simulink model "X31dynamics_03_controller_NDI_MG"  (R2014b)
settings: Solver=ode45  StartTime=0.0  StopTime=30  FixedStep=0.01  RelTol=1e-3
InitFcn:
  | X31dynamics_03_controller_NDI_init
values from neighbouring files (symbols this model uses):
  X31_controller = evalin('base','X31_controller')    [X31dynamics_03_controller_MG_iter_3_2_9_10.m]
undefined symbols (not defined in the file or in its folder): sigbuilder_block, X31_initC, X31_MnvrGen
libraries: simulink x17, QuaternionLib x3
(part 1 of 2)
settings Model: Creator=Ewing  LastModifiedBy=5909
settings SolverCC: AlgebraicLoopSolver=LineSearch
settings DataIOCC: SaveOutput=off  SaveTime=off
settings OptimizationCC: InlineParams=on  InlineInvariantSignals=on  EfficientFloat2IntCast=on
settings DebuggingCC: UnderspecifiedInitializationDetection=Classic  MergeDetectMultiDrivingBlocksExec=none  UniqueDataStoreMsg=error  StateNameClashWarn=warning
settings ModelReferenceCC: ModelReferencePassRootInputsByReference=off

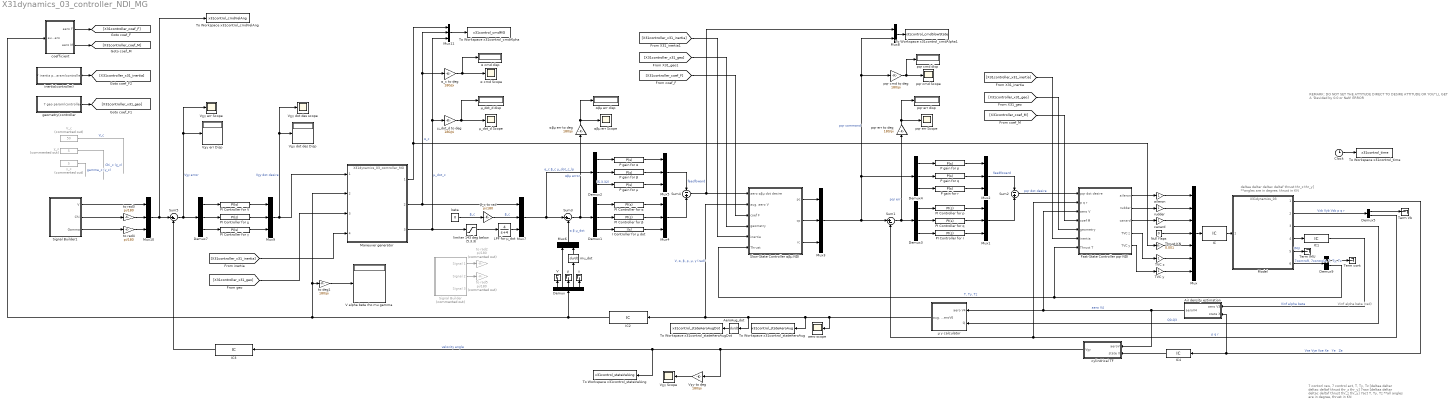
== system X31dynamics_03_controller_NDI_MG ==
  note: REMARK: DO NOT SET THE ATTITUDE DIRECT TO DESIRE ATTITUDE
      | OR YOU"LL GET A 'Devided by 0.0 or NaN' ERROR
  note: deltaa deltar deltac deltaf thrust thr_z thr_y]
      | **angles are in degree, thrust in KN
  note: Vinf alpha beta (rad)
  note: 7 contorl raw, 7 control act, T, Ty, Tz
      | [deltaa deltar deltac deltaf thrust thr_z thr_y] 7raw
      | [deltaa deltar deltac deltaf thrust thr_z thr_y] 7act
      | T, Ty, Tz
      | **all angles are in degree, thrust in KN
  AeroAug_dot : Derivative
  Air density estimation : Subsystem
  Clock : Clock
  Demux : Demux  Outputs=[1 2 1 1 1]
  Demux{1..4,7} (5 alike) : Demux  Outputs=3
  Demux5 : Demux  Outputs=[3 3]
  Demux9 : Demux  Outputs=[14 3]
  Fast-State Controller pqr NDI : Subsystem
  I Controller for μ dot : simulink/Continuous/PID Controller  Controller=I  TimeDomain=Continuous-time  SampleTime=-1  IntegratorMethod=Forward Euler  FilterMethod=Forward Euler  Form=Parallel  P=1  I=X31_controller.gains.slow_st.mu_dot.I_gain  D=0  N=100  InitialConditionSource=internal  InitialConditionForIntegrator=0  InitialConditionForFilter=0  ExternalReset=none  LimitOutput=off  UpperSaturationLimit=inf  LowerSaturationLimit=-inf  LinearizeAsGain=on  AntiWindupMode=none  Kb=1  TrackingMode=off  Kt=1  PParamMin=[]  PParamMax=[]  IParamMin=[]  IParamMax=[]  DParamMin=[]  DParamMax=[]  NParamMin=[]  NParamMax=[]  KbParamMin=[]  KbParamMax=[]  KtParamMin=[]  KtParamMax=[]  POutMin=[]  POutMax=[]  IOutMin=[]  IOutMax=[]  DOutMin=[]  DOutMax=[]  NOutMin=[]  NOutMax=[]  KbOutMin=[]  KbOutMax=[]  KtOutMin=[]  KtOutMax=[]  IntegratorOutMin=[]  IntegratorOutMax=[]  FilterOutMin=[]  FilterOutMax=[]  SumOutMin=[]  SumOutMax=[]  SumI1OutMin=[]  SumI1OutMax=[]  SumI2OutMin=[]  SumI2OutMax=[]  SumI3OutMin=[]  SumI3OutMax=[]  SumDOutMin=[]  SumDOutMax=[]  SaturationOutMin=[]  SaturationOutMax=[]  IntegratorContinuousStateAttributes=''  IntegratorStateMustResolveToSignalObject=off  IntegratorRTWStateStorageClass=Auto  FilterContinuousStateAttributes=''  FilterStateMustResolveToSignalObject=off  FilterRTWStateStorageClass=Auto  DifferentiatorICPrevScaledInput=0  DifferentiatorOutMin=[]  DifferentiatorOutMax=[]  UseFilter=on
  IC : InitialCondition  Value=[ 0.0001 0.0001 0.0001 0.0001 X31_initC.thrust 0.0001 0.0001]
  IC1 : InitialCondition  Value=[50 0.01 0.01]
  IC2 : InitialCondition  Value=[50 5 0 1.23 0 0]
  IC3 : InitialCondition  Value=[50 0 0]
  IC4 : InitialCondition  Value=[50 0 0 0.1 0.1 -0.1]
  LPF for μ_dot : TransferFcn  Numerator=[4]  Denominator=[1 4]
  Maneuver generator : ModelReference  ModelNameDialog=X31dynamics_03_controller_MG.slx  SimulationMode=Normal  ModelReferenceVersion=1.4  CopyOfModelName=X31dynamics_03_controller_MG.slx  DefaultDataLogging=on
  Model : ModelReference  ModelNameDialog=X31dynamics_03.slx  SimulationMode=Normal  ModelReferenceVersion=1.305  CopyOfModelName=X31dynamics_03.slx  DefaultDataLogging=on
  Mux : Mux  Inputs=7
  Mux{1..5,7,9..11} (9 alike) : Mux  Inputs=3
  Mux6 : Mux  Inputs=2
  Mux8 : Mux  Inputs=2
  Null flaps : Constant  Value=0
  P gain for p : simulink/Continuous/PID Controller  Controller=P  TimeDomain=Continuous-time  SampleTime=-1  IntegratorMethod=Forward Euler  FilterMethod=Forward Euler  Form=Parallel  P=X31_controller.gains.fast_st.p.ff_gain  I=1  D=0  N=100  InitialConditionSource=internal  InitialConditionForIntegrator=0  InitialConditionForFilter=0  ExternalReset=none  LimitOutput=off  UpperSaturationLimit=inf  LowerSaturationLimit=-inf  LinearizeAsGain=on  AntiWindupMode=none  Kb=1  TrackingMode=off  Kt=1  PParamMin=[]  PParamMax=[]  IParamMin=[]  IParamMax=[]  DParamMin=[]  DParamMax=[]  NParamMin=[]  NParamMax=[]  KbParamMin=[]  KbParamMax=[]  KtParamMin=[]  KtParamMax=[]  POutMin=[]  POutMax=[]  IOutMin=[]  IOutMax=[]  DOutMin=[]  DOutMax=[]  NOutMin=[]  NOutMax=[]  KbOutMin=[]  KbOutMax=[]  KtOutMin=[]  KtOutMax=[]  IntegratorOutMin=[]  IntegratorOutMax=[]  FilterOutMin=[]  FilterOutMax=[]  SumOutMin=[]  SumOutMax=[]  SumI1OutMin=[]  SumI1OutMax=[]  SumI2OutMin=[]  SumI2OutMax=[]  SumI3OutMin=[]  SumI3OutMax=[]  SumDOutMin=[]  SumDOutMax=[]  SaturationOutMin=[]  SaturationOutMax=[]  IntegratorContinuousStateAttributes=''  IntegratorStateMustResolveToSignalObject=off  IntegratorRTWStateStorageClass=Auto  FilterContinuousStateAttributes=''  FilterStateMustResolveToSignalObject=off  FilterRTWStateStorageClass=Auto  DifferentiatorICPrevScaledInput=0  DifferentiatorOutMin=[]  DifferentiatorOutMax=[]  UseFilter=on
  P gain for q : simulink/Continuous/PID Controller  Controller=P  TimeDomain=Continuous-time  SampleTime=-1  IntegratorMethod=Forward Euler  FilterMethod=Forward Euler  Form=Parallel  P=X31_controller.gains.fast_st.q.ff_gain  I=1  D=0  N=100  InitialConditionSource=internal  InitialConditionForIntegrator=0  InitialConditionForFilter=0  ExternalReset=none  LimitOutput=off  UpperSaturationLimit=inf  LowerSaturationLimit=-inf  LinearizeAsGain=on  AntiWindupMode=none  Kb=1  TrackingMode=off  Kt=1  PParamMin=[]  PParamMax=[]  IParamMin=[]  IParamMax=[]  DParamMin=[]  DParamMax=[]  NParamMin=[]  NParamMax=[]  KbParamMin=[]  KbParamMax=[]  KtParamMin=[]  KtParamMax=[]  POutMin=[]  POutMax=[]  IOutMin=[]  IOutMax=[]  DOutMin=[]  DOutMax=[]  NOutMin=[]  NOutMax=[]  KbOutMin=[]  KbOutMax=[]  KtOutMin=[]  KtOutMax=[]  IntegratorOutMin=[]  IntegratorOutMax=[]  FilterOutMin=[]  FilterOutMax=[]  SumOutMin=[]  SumOutMax=[]  SumI1OutMin=[]  SumI1OutMax=[]  SumI2OutMin=[]  SumI2OutMax=[]  SumI3OutMin=[]  SumI3OutMax=[]  SumDOutMin=[]  SumDOutMax=[]  SaturationOutMin=[]  SaturationOutMax=[]  IntegratorContinuousStateAttributes=''  IntegratorStateMustResolveToSignalObject=off  IntegratorRTWStateStorageClass=Auto  FilterContinuousStateAttributes=''  FilterStateMustResolveToSignalObject=off  FilterRTWStateStorageClass=Auto  DifferentiatorICPrevScaledInput=0  DifferentiatorOutMin=[]  DifferentiatorOutMax=[]  UseFilter=on
  P gain for r : simulink/Continuous/PID Controller  Controller=P  TimeDomain=Continuous-time  SampleTime=-1  IntegratorMethod=Forward Euler  FilterMethod=Forward Euler  Form=Parallel  P=X31_controller.gains.fast_st.r.ff_gain  I=1  D=0  N=100  InitialConditionSource=internal  InitialConditionForIntegrator=0  InitialConditionForFilter=0  ExternalReset=none  LimitOutput=off  UpperSaturationLimit=inf  LowerSaturationLimit=-inf  LinearizeAsGain=on  AntiWindupMode=none  Kb=1  TrackingMode=off  Kt=1  PParamMin=[]  PParamMax=[]  IParamMin=[]  IParamMax=[]  DParamMin=[]  DParamMax=[]  NParamMin=[]  NParamMax=[]  KbParamMin=[]  KbParamMax=[]  KtParamMin=[]  KtParamMax=[]  POutMin=[]  POutMax=[]  IOutMin=[]  IOutMax=[]  DOutMin=[]  DOutMax=[]  NOutMin=[]  NOutMax=[]  KbOutMin=[]  KbOutMax=[]  KtOutMin=[]  KtOutMax=[]  IntegratorOutMin=[]  IntegratorOutMax=[]  FilterOutMin=[]  FilterOutMax=[]  SumOutMin=[]  SumOutMax=[]  SumI1OutMin=[]  SumI1OutMax=[]  SumI2OutMin=[]  SumI2OutMax=[]  SumI3OutMin=[]  SumI3OutMax=[]  SumDOutMin=[]  SumDOutMax=[]  SaturationOutMin=[]  SaturationOutMax=[]  IntegratorContinuousStateAttributes=''  IntegratorStateMustResolveToSignalObject=off  IntegratorRTWStateStorageClass=Auto  FilterContinuousStateAttributes=''  FilterStateMustResolveToSignalObject=off  FilterRTWStateStorageClass=Auto  DifferentiatorICPrevScaledInput=0  DifferentiatorOutMin=[]  DifferentiatorOutMax=[]  UseFilter=on
  P gain for α : simulink/Continuous/PID Controller  Controller=P  TimeDomain=Continuous-time  SampleTime=-1  IntegratorMethod=Forward Euler  FilterMethod=Forward Euler  Form=Parallel  P=X31_controller.gains.slow_st.alpha.ff_gain  I=1  D=0  N=100  InitialConditionSource=internal  InitialConditionForIntegrator=0  InitialConditionForFilter=0  ExternalReset=none  LimitOutput=off  UpperSaturationLimit=inf  LowerSaturationLimit=-inf  LinearizeAsGain=on  AntiWindupMode=none  Kb=1  TrackingMode=off  Kt=1  PParamMin=[]  PParamMax=[]  IParamMin=[]  IParamMax=[]  DParamMin=[]  DParamMax=[]  NParamMin=[]  NParamMax=[]  KbParamMin=[]  KbParamMax=[]  KtParamMin=[]  KtParamMax=[]  POutMin=[]  POutMax=[]  IOutMin=[]  IOutMax=[]  DOutMin=[]  DOutMax=[]  NOutMin=[]  NOutMax=[]  KbOutMin=[]  KbOutMax=[]  KtOutMin=[]  KtOutMax=[]  IntegratorOutMin=[]  IntegratorOutMax=[]  FilterOutMin=[]  FilterOutMax=[]  SumOutMin=[]  SumOutMax=[]  SumI1OutMin=[]  SumI1OutMax=[]  SumI2OutMin=[]  SumI2OutMax=[]  SumI3OutMin=[]  SumI3OutMax=[]  SumDOutMin=[]  SumDOutMax=[]  SaturationOutMin=[]  SaturationOutMax=[]  IntegratorContinuousStateAttributes=''  IntegratorStateMustResolveToSignalObject=off  IntegratorRTWStateStorageClass=Auto  FilterContinuousStateAttributes=''  FilterStateMustResolveToSignalObject=off  FilterRTWStateStorageClass=Auto  DifferentiatorICPrevScaledInput=0  DifferentiatorOutMin=[]  DifferentiatorOutMax=[]  UseFilter=on
  P gain for β : simulink/Continuous/PID Controller  Controller=P  TimeDomain=Continuous-time  SampleTime=-1  IntegratorMethod=Forward Euler  FilterMethod=Forward Euler  Form=Parallel  P=X31_controller.gains.slow_st.beta.ff_gain  I=1  D=0  N=100  InitialConditionSource=internal  InitialConditionForIntegrator=0  InitialConditionForFilter=0  ExternalReset=none  LimitOutput=off  UpperSaturationLimit=inf  LowerSaturationLimit=-inf  LinearizeAsGain=on  AntiWindupMode=none  Kb=1  TrackingMode=off  Kt=1  PParamMin=[]  PParamMax=[]  IParamMin=[]  IParamMax=[]  DParamMin=[]  DParamMax=[]  NParamMin=[]  NParamMax=[]  KbParamMin=[]  KbParamMax=[]  KtParamMin=[]  KtParamMax=[]  POutMin=[]  POutMax=[]  IOutMin=[]  IOutMax=[]  DOutMin=[]  DOutMax=[]  NOutMin=[]  NOutMax=[]  KbOutMin=[]  KbOutMax=[]  KtOutMin=[]  KtOutMax=[]  IntegratorOutMin=[]  IntegratorOutMax=[]  FilterOutMin=[]  FilterOutMax=[]  SumOutMin=[]  SumOutMax=[]  SumI1OutMin=[]  SumI1OutMax=[]  SumI2OutMin=[]  SumI2OutMax=[]  SumI3OutMin=[]  SumI3OutMax=[]  SumDOutMin=[]  SumDOutMax=[]  SaturationOutMin=[]  SaturationOutMax=[]  IntegratorContinuousStateAttributes=''  IntegratorStateMustResolveToSignalObject=off  IntegratorRTWStateStorageClass=Auto  FilterContinuousStateAttributes=''  FilterStateMustResolveToSignalObject=off  FilterRTWStateStorageClass=Auto  DifferentiatorICPrevScaledInput=0  DifferentiatorOutMin=[]  DifferentiatorOutMax=[]  UseFilter=on
  P gain for μ : simulink/Continuous/PID Controller  Controller=P  TimeDomain=Continuous-time  SampleTime=-1  IntegratorMethod=Forward Euler  FilterMethod=Forward Euler  Form=Parallel  P=X31_controller.gains.slow_st.mu_dot.ff_gain  I=1  D=0  N=100  InitialConditionSource=internal  InitialConditionForIntegrator=0  InitialConditionForFilter=0  ExternalReset=none  LimitOutput=off  UpperSaturationLimit=inf  LowerSaturationLimit=-inf  LinearizeAsGain=on  AntiWindupMode=none  Kb=1  TrackingMode=off  Kt=1  PParamMin=[]  PParamMax=[]  IParamMin=[]  IParamMax=[]  DParamMin=[]  DParamMax=[]  NParamMin=[]  NParamMax=[]  KbParamMin=[]  KbParamMax=[]  KtParamMin=[]  KtParamMax=[]  POutMin=[]  POutMax=[]  IOutMin=[]  IOutMax=[]  DOutMin=[]  DOutMax=[]  NOutMin=[]  NOutMax=[]  KbOutMin=[]  KbOutMax=[]  KtOutMin=[]  KtOutMax=[]  IntegratorOutMin=[]  IntegratorOutMax=[]  FilterOutMin=[]  FilterOutMax=[]  SumOutMin=[]  SumOutMax=[]  SumI1OutMin=[]  SumI1OutMax=[]  SumI2OutMin=[]  SumI2OutMax=[]  SumI3OutMin=[]  SumI3OutMax=[]  SumDOutMin=[]  SumDOutMax=[]  SaturationOutMin=[]  SaturationOutMax=[]  IntegratorContinuousStateAttributes=''  IntegratorStateMustResolveToSignalObject=off  IntegratorRTWStateStorageClass=Auto  FilterContinuousStateAttributes=''  FilterStateMustResolveToSignalObject=off  FilterRTWStateStorageClass=Auto  DifferentiatorICPrevScaledInput=0  DifferentiatorOutMin=[]  DifferentiatorOutMax=[]  UseFilter=on
  PI Controller for V : simulink/Continuous/PID Controller  Controller=PI  TimeDomain=Continuous-time  SampleTime=-1  IntegratorMethod=Forward Euler  FilterMethod=Forward Euler  Form=Parallel  P=X31_MnvrGen.gains.vel.P_gain  I=X31_MnvrGen.gains.vel.I_gain  D=0  N=100  InitialConditionSource=internal  InitialConditionForIntegrator=0  InitialConditionForFilter=0  ExternalReset=none  LimitOutput=off  UpperSaturationLimit=inf  LowerSaturationLimit=-inf  LinearizeAsGain=on  AntiWindupMode=none  Kb=1  TrackingMode=off  Kt=1  PParamMin=[]  PParamMax=[]  IParamMin=[]  IParamMax=[]  DParamMin=[]  DParamMax=[]  NParamMin=[]  NParamMax=[]  KbParamMin=[]  KbParamMax=[]  KtParamMin=[]  KtParamMax=[]  POutMin=[]  POutMax=[]  IOutMin=[]  IOutMax=[]  DOutMin=[]  DOutMax=[]  NOutMin=[]  NOutMax=[]  KbOutMin=[]  KbOutMax=[]  KtOutMin=[]  KtOutMax=[]  IntegratorOutMin=[]  IntegratorOutMax=[]  FilterOutMin=[]  FilterOutMax=[]  SumOutMin=[]  SumOutMax=[]  SumI1OutMin=[]  SumI1OutMax=[]  SumI2OutMin=[]  SumI2OutMax=[]  SumI3OutMin=[]  SumI3OutMax=[]  SumDOutMin=[]  SumDOutMax=[]  SaturationOutMin=[]  SaturationOutMax=[]  IntegratorContinuousStateAttributes=''  IntegratorStateMustResolveToSignalObject=off  IntegratorRTWStateStorageClass=Auto  FilterContinuousStateAttributes=''  FilterStateMustResolveToSignalObject=off  FilterRTWStateStorageClass=Auto  DifferentiatorICPrevScaledInput=0  DifferentiatorOutMin=[]  DifferentiatorOutMax=[]  UseFilter=on
  PI Controller for p : simulink/Continuous/PID Controller  Controller=PI  TimeDomain=Continuous-time  SampleTime=-1  IntegratorMethod=Forward Euler  FilterMethod=Forward Euler  Form=Parallel  P=X31_controller.gains.fast_st.p.P_gain  I=X31_controller.gains.fast_st.p.I_gain  D=0  N=100  InitialConditionSource=internal  InitialConditionForIntegrator=0  InitialConditionForFilter=0  ExternalReset=none  LimitOutput=off  UpperSaturationLimit=inf  LowerSaturationLimit=-inf  LinearizeAsGain=on  AntiWindupMode=none  Kb=1  TrackingMode=off  Kt=1  PParamMin=[]  PParamMax=[]  IParamMin=[]  IParamMax=[]  DParamMin=[]  DParamMax=[]  NParamMin=[]  NParamMax=[]  KbParamMin=[]  KbParamMax=[]  KtParamMin=[]  KtParamMax=[]  POutMin=[]  POutMax=[]  IOutMin=[]  IOutMax=[]  DOutMin=[]  DOutMax=[]  NOutMin=[]  NOutMax=[]  KbOutMin=[]  KbOutMax=[]  KtOutMin=[]  KtOutMax=[]  IntegratorOutMin=[]  IntegratorOutMax=[]  FilterOutMin=[]  FilterOutMax=[]  SumOutMin=[]  SumOutMax=[]  SumI1OutMin=[]  SumI1OutMax=[]  SumI2OutMin=[]  SumI2OutMax=[]  SumI3OutMin=[]  SumI3OutMax=[]  SumDOutMin=[]  SumDOutMax=[]  SaturationOutMin=[]  SaturationOutMax=[]  IntegratorContinuousStateAttributes=''  IntegratorStateMustResolveToSignalObject=off  IntegratorRTWStateStorageClass=Auto  FilterContinuousStateAttributes=''  FilterStateMustResolveToSignalObject=off  FilterRTWStateStorageClass=Auto  DifferentiatorICPrevScaledInput=0  DifferentiatorOutMin=[]  DifferentiatorOutMax=[]  UseFilter=on
  PI Controller for q : simulink/Continuous/PID Controller  Controller=PI  TimeDomain=Continuous-time  SampleTime=-1  IntegratorMethod=Forward Euler  FilterMethod=Forward Euler  Form=Parallel  P=X31_controller.gains.fast_st.q.P_gain  I=X31_controller.gains.fast_st.q.I_gain  D=0  N=100  InitialConditionSource=internal  InitialConditionForIntegrator=0  InitialConditionForFilter=0  ExternalReset=none  LimitOutput=off  UpperSaturationLimit=inf  LowerSaturationLimit=-inf  LinearizeAsGain=on  AntiWindupMode=none  Kb=1  TrackingMode=off  Kt=1  PParamMin=[]  PParamMax=[]  IParamMin=[]  IParamMax=[]  DParamMin=[]  DParamMax=[]  NParamMin=[]  NParamMax=[]  KbParamMin=[]  KbParamMax=[]  KtParamMin=[]  KtParamMax=[]  POutMin=[]  POutMax=[]  IOutMin=[]  IOutMax=[]  DOutMin=[]  DOutMax=[]  NOutMin=[]  NOutMax=[]  KbOutMin=[]  KbOutMax=[]  KtOutMin=[]  KtOutMax=[]  IntegratorOutMin=[]  IntegratorOutMax=[]  FilterOutMin=[]  FilterOutMax=[]  SumOutMin=[]  SumOutMax=[]  SumI1OutMin=[]  SumI1OutMax=[]  SumI2OutMin=[]  SumI2OutMax=[]  SumI3OutMin=[]  SumI3OutMax=[]  SumDOutMin=[]  SumDOutMax=[]  SaturationOutMin=[]  SaturationOutMax=[]  IntegratorContinuousStateAttributes=''  IntegratorStateMustResolveToSignalObject=off  IntegratorRTWStateStorageClass=Auto  FilterContinuousStateAttributes=''  FilterStateMustResolveToSignalObject=off  FilterRTWStateStorageClass=Auto  DifferentiatorICPrevScaledInput=0  DifferentiatorOutMin=[]  DifferentiatorOutMax=[]  UseFilter=on
  PI Controller for r : simulink/Continuous/PID Controller  Controller=PI  TimeDomain=Continuous-time  SampleTime=-1  IntegratorMethod=Forward Euler  FilterMethod=Forward Euler  Form=Parallel  P=X31_controller.gains.fast_st.r.P_gain  I=X31_controller.gains.fast_st.r.I_gain  D=0  N=100  InitialConditionSource=internal  InitialConditionForIntegrator=0  InitialConditionForFilter=0  ExternalReset=none  LimitOutput=off  UpperSaturationLimit=inf  LowerSaturationLimit=-inf  LinearizeAsGain=on  AntiWindupMode=none  Kb=1  TrackingMode=off  Kt=1  PParamMin=[]  PParamMax=[]  IParamMin=[]  IParamMax=[]  DParamMin=[]  DParamMax=[]  NParamMin=[]  NParamMax=[]  KbParamMin=[]  KbParamMax=[]  KtParamMin=[]  KtParamMax=[]  POutMin=[]  POutMax=[]  IOutMin=[]  IOutMax=[]  DOutMin=[]  DOutMax=[]  NOutMin=[]  NOutMax=[]  KbOutMin=[]  KbOutMax=[]  KtOutMin=[]  KtOutMax=[]  IntegratorOutMin=[]  IntegratorOutMax=[]  FilterOutMin=[]  FilterOutMax=[]  SumOutMin=[]  SumOutMax=[]  SumI1OutMin=[]  SumI1OutMax=[]  SumI2OutMin=[]  SumI2OutMax=[]  SumI3OutMin=[]  SumI3OutMax=[]  SumDOutMin=[]  SumDOutMax=[]  SaturationOutMin=[]  SaturationOutMax=[]  IntegratorContinuousStateAttributes=''  IntegratorStateMustResolveToSignalObject=off  IntegratorRTWStateStorageClass=Auto  FilterContinuousStateAttributes=''  FilterStateMustResolveToSignalObject=off  FilterRTWStateStorageClass=Auto  DifferentiatorICPrevScaledInput=0  DifferentiatorOutMin=[]  DifferentiatorOutMax=[]  UseFilter=on
  PI Controller for α : simulink/Continuous/PID Controller  Controller=PI  TimeDomain=Continuous-time  SampleTime=-1  IntegratorMethod=Forward Euler  FilterMethod=Forward Euler  Form=Parallel  P=X31_controller.gains.slow_st.alpha.P_gain  I=X31_controller.gains.slow_st.alpha.I_gain  D=0  N=100  InitialConditionSource=internal  InitialConditionForIntegrator=0  InitialConditionForFilter=0  ExternalReset=none  LimitOutput=off  UpperSaturationLimit=inf  LowerSaturationLimit=-inf  LinearizeAsGain=on  AntiWindupMode=none  Kb=1  TrackingMode=off  Kt=1  PParamMin=[]  PParamMax=[]  IParamMin=[]  IParamMax=[]  DParamMin=[]  DParamMax=[]  NParamMin=[]  NParamMax=[]  KbParamMin=[]  KbParamMax=[]  KtParamMin=[]  KtParamMax=[]  POutMin=[]  POutMax=[]  IOutMin=[]  IOutMax=[]  DOutMin=[]  DOutMax=[]  NOutMin=[]  NOutMax=[]  KbOutMin=[]  KbOutMax=[]  KtOutMin=[]  KtOutMax=[]  IntegratorOutMin=[]  IntegratorOutMax=[]  FilterOutMin=[]  FilterOutMax=[]  SumOutMin=[]  SumOutMax=[]  SumI1OutMin=[]  SumI1OutMax=[]  SumI2OutMin=[]  SumI2OutMax=[]  SumI3OutMin=[]  SumI3OutMax=[]  SumDOutMin=[]  SumDOutMax=[]  SaturationOutMin=[]  SaturationOutMax=[]  IntegratorContinuousStateAttributes=''  IntegratorStateMustResolveToSignalObject=off  IntegratorRTWStateStorageClass=Auto  FilterContinuousStateAttributes=''  FilterStateMustResolveToSignalObject=off  FilterRTWStateStorageClass=Auto  DifferentiatorICPrevScaledInput=0  DifferentiatorOutMin=[]  DifferentiatorOutMax=[]  UseFilter=on
  PI Controller for β : simulink/Continuous/PID Controller  Controller=PI  TimeDomain=Continuous-time  SampleTime=-1  IntegratorMethod=Forward Euler  FilterMethod=Forward Euler  Form=Parallel  P=X31_controller.gains.slow_st.beta.P_gain  I=X31_controller.gains.slow_st.beta.I_gain  D=0  N=100  InitialConditionSource=internal  InitialConditionForIntegrator=0  InitialConditionForFilter=0  ExternalReset=none  LimitOutput=off  UpperSaturationLimit=inf  LowerSaturationLimit=-inf  LinearizeAsGain=on  AntiWindupMode=none  Kb=1  TrackingMode=off  Kt=1  PParamMin=[]  PParamMax=[]  IParamMin=[]  IParamMax=[]  DParamMin=[]  DParamMax=[]  NParamMin=[]  NParamMax=[]  KbParamMin=[]  KbParamMax=[]  KtParamMin=[]  KtParamMax=[]  POutMin=[]  POutMax=[]  IOutMin=[]  IOutMax=[]  DOutMin=[]  DOutMax=[]  NOutMin=[]  NOutMax=[]  KbOutMin=[]  KbOutMax=[]  KtOutMin=[]  KtOutMax=[]  IntegratorOutMin=[]  IntegratorOutMax=[]  FilterOutMin=[]  FilterOutMax=[]  SumOutMin=[]  SumOutMax=[]  SumI1OutMin=[]  SumI1OutMax=[]  SumI2OutMin=[]  SumI2OutMax=[]  SumI3OutMin=[]  SumI3OutMax=[]  SumDOutMin=[]  SumDOutMax=[]  SaturationOutMin=[]  SaturationOutMax=[]  IntegratorContinuousStateAttributes=''  IntegratorStateMustResolveToSignalObject=off  IntegratorRTWStateStorageClass=Auto  FilterContinuousStateAttributes=''  FilterStateMustResolveToSignalObject=off  FilterRTWStateStorageClass=Auto  DifferentiatorICPrevScaledInput=0  DifferentiatorOutMin=[]  DifferentiatorOutMax=[]  UseFilter=on
  PI Controller for γ : simulink/Continuous/PID Controller  Controller=PI  TimeDomain=Continuous-time  SampleTime=-1  IntegratorMethod=Forward Euler  FilterMethod=Forward Euler  Form=Parallel  P=X31_MnvrGen.gains.gamma.P_gain  I=X31_MnvrGen.gains.gamma.P_gain  D=0  N=100  InitialConditionSource=internal  InitialConditionForIntegrator=0  InitialConditionForFilter=0  ExternalReset=none  LimitOutput=off  UpperSaturationLimit=inf  LowerSaturationLimit=-inf  LinearizeAsGain=on  AntiWindupMode=none  Kb=1  TrackingMode=off  Kt=1  PParamMin=[]  PParamMax=[]  IParamMin=[]  IParamMax=[]  DParamMin=[]  DParamMax=[]  NParamMin=[]  NParamMax=[]  KbParamMin=[]  KbParamMax=[]  KtParamMin=[]  KtParamMax=[]  POutMin=[]  POutMax=[]  IOutMin=[]  IOutMax=[]  DOutMin=[]  DOutMax=[]  NOutMin=[]  NOutMax=[]  KbOutMin=[]  KbOutMax=[]  KtOutMin=[]  KtOutMax=[]  IntegratorOutMin=[]  IntegratorOutMax=[]  FilterOutMin=[]  FilterOutMax=[]  SumOutMin=[]  SumOutMax=[]  SumI1OutMin=[]  SumI1OutMax=[]  SumI2OutMin=[]  SumI2OutMax=[]  SumI3OutMin=[]  SumI3OutMax=[]  SumDOutMin=[]  SumDOutMax=[]  SaturationOutMin=[]  SaturationOutMax=[]  IntegratorContinuousStateAttributes=''  IntegratorStateMustResolveToSignalObject=off  IntegratorRTWStateStorageClass=Auto  FilterContinuousStateAttributes=''  FilterStateMustResolveToSignalObject=off  FilterRTWStateStorageClass=Auto  DifferentiatorICPrevScaledInput=0  DifferentiatorOutMin=[]  DifferentiatorOutMax=[]  UseFilter=on
  PI Controller for χ : simulink/Continuous/PID Controller  Controller=PI  TimeDomain=Continuous-time  SampleTime=-1  IntegratorMethod=Forward Euler  FilterMethod=Forward Euler  Form=Parallel  P=X31_MnvrGen.gains.chi.P_gain  I=X31_MnvrGen.gains.chi.I_gain  D=0  N=100  InitialConditionSource=internal  InitialConditionForIntegrator=0  InitialConditionForFilter=0  ExternalReset=none  LimitOutput=off  UpperSaturationLimit=inf  LowerSaturationLimit=-inf  LinearizeAsGain=on  AntiWindupMode=none  Kb=1  TrackingMode=off  Kt=1  PParamMin=[]  PParamMax=[]  IParamMin=[]  IParamMax=[]  DParamMin=[]  DParamMax=[]  NParamMin=[]  NParamMax=[]  KbParamMin=[]  KbParamMax=[]  KtParamMin=[]  KtParamMax=[]  POutMin=[]  POutMax=[]  IOutMin=[]  IOutMax=[]  DOutMin=[]  DOutMax=[]  NOutMin=[]  NOutMax=[]  KbOutMin=[]  KbOutMax=[]  KtOutMin=[]  KtOutMax=[]  IntegratorOutMin=[]  IntegratorOutMax=[]  FilterOutMin=[]  FilterOutMax=[]  SumOutMin=[]  SumOutMax=[]  SumI1OutMin=[]  SumI1OutMax=[]  SumI2OutMin=[]  SumI2OutMax=[]  SumI3OutMin=[]  SumI3OutMax=[]  SumDOutMin=[]  SumDOutMax=[]  SaturationOutMin=[]  SaturationOutMax=[]  IntegratorContinuousStateAttributes=''  IntegratorStateMustResolveToSignalObject=off  IntegratorRTWStateStorageClass=Auto  FilterContinuousStateAttributes=''  FilterStateMustResolveToSignalObject=off  FilterRTWStateStorageClass=Auto  DifferentiatorICPrevScaledInput=0  DifferentiatorOutMin=[]  DifferentiatorOutMax=[]  UseFilter=on
  Signal Builder : Subsystem  Tag=STV Subsys  Commented=on  LoadFcn=sigbuilder_block('load');  StartFcn=sigbuilder_block('start');  StopFcn=sigbuilder_block('stop');  ClipboardFcn=sigbuilder_block('clipboard');  mask(Sigbuilder block){}
      mask help: Simulink:masks:SigbuilderBlock_MD
      mask init:
      | if ~strcmp(get_param(bdroot(gcbh),'SimulationStatus'),'stopped') tuvar = sigbuilder_block('maskInit'); end
      settings: CopyFcn=sigbuilder_block('copy');  DeleteFcn=sigbuilder_block('delete');  ModelCloseFcn=sigbuilder_block('modelClose');  PreSaveFcn=sigbuilder_block('preSave');  PauseFcn=sigbuilder_block('pause');  ContinueFcn=sigbuilder_block('continue');  NameChangeFcn=sigbuilder_block('namechange');  OpenFcn=sigbuilder_block('open',[437.6 199.2 550.4 400 ]);  CloseFcn=sigbuilder_block('close');
      mask Display: plot(0, 0, 100, 100,[2, 2, 32, 32, 2], [68, 8, 8, 68, 68],[32, 2], [38, 38], [32, 19, 2],[53, 60, 44], [32, 17, 17, 2],[16, 16, 31, 31]);txt = getActiveGroup(gcbh);text(2, 100, txt,'verticalAlignment', 'top');
  Signal Builder1 : Subsystem  Tag=STV Subsys  LoadFcn=sigbuilder_block('load');  StartFcn=sigbuilder_block('start');  StopFcn=sigbuilder_block('stop');  ClipboardFcn=sigbuilder_block('clipboard');  mask(Sigbuilder block){}
      mask help: Simulink:masks:SigbuilderBlock_MD
      mask init:
      | if ~strcmp(get_param(bdroot(gcbh),'SimulationStatus'),'stopped') tuvar = sigbuilder_block('maskInit'); end
      settings: CopyFcn=sigbuilder_block('copy');  DeleteFcn=sigbuilder_block('delete');  ModelCloseFcn=sigbuilder_block('modelClose');  PreSaveFcn=sigbuilder_block('preSave');  PauseFcn=sigbuilder_block('pause');  ContinueFcn=sigbuilder_block('continue');  NameChangeFcn=sigbuilder_block('namechange');  OpenFcn=sigbuilder_block('open',[437.6 199.2 550.4 400 ]);  CloseFcn=sigbuilder_block('close');
      mask Display: plot(0, 0, 100, 100,[2, 2, 32, 32, 2], [68, 8, 8, 68, 68],[32, 2], [38, 38], [32, 19, 2],[53, 60, 44], [32, 17, 17, 2],[16, 16, 31, 31]);txt = getActiveGroup(gcbh);text(2, 100, txt,'verticalAlignment', 'top');
  Slow-State Controller αβμ NDI : Subsystem
  Sum1 : Sum  Inputs=|+-
  Sum2 : Sum  Inputs=-|+
  Sum3 : Sum  Inputs=|+-
  Sum4 : Sum  Inputs=-|+
  Sum5 : Sum  Inputs=|+-
  TVC y : Gain
  TVC z : Gain
  Term IMU : Terminator
  Term Vb : Terminator
  Term cont : Terminator
  Thrust KN : Gain  Gain=0.001
  To Workspace x31control_cmdAlpha : ToWorkspace  VariableName=x31control_cmdMG  SaveFormat=Timeseries  SampleTime=-1
  To Workspace x31control_cmdAlpha1 : ToWorkspace  VariableName=x31control_cmdSlowState  SaveFormat=Timeseries  SampleTime=-1
  To Workspace x31control_cmdVelAng : ToWorkspace  VariableName=x31control_cmdVelAng  SaveFormat=Timeseries  SampleTime=-1
  To Workspace x31control_stateAeroAug : ToWorkspace  VariableName=x31control_stateAeroAug  SaveFormat=Timeseries  SampleTime=-1
  To Workspace x31control_stateAeroAugDot : ToWorkspace  VariableName=x31control_stateAeroAugDot  SaveFormat=Timeseries  SampleTime=-1
  To Workspace x31control_stateVelAng : ToWorkspace  VariableName=x31control_stateVelAng  SaveFormat=Timeseries  SampleTime=-1
  To Workspace x31control_time : ToWorkspace  VariableName=x31control_time  SaveFormat=Timeseries  SampleTime=-1
  V : Terminator
  V alpha beta rho mu gamma : Display
  V_c : Constant  Commented=on  Value=50
  Vχγ Scope : Scope
      settings: ShowLegends=on  TimeRange=30  YMin=-1000  YMax=6000  SaveName=ScopeData18
  Vχγ dot des Disp : Display
  Vχγ dot des scope : Scope
      settings: TickLabels=on  ShowLegends=on  SaveName=ScopeData15
  Vχγ err Disp : Display
  Vχγ err Scope : Scope
      settings: TimeRange=3.005065038857998  YMin=2.02995391705069  YMax=6.02995391705069  SaveName=ScopeData14
  Vχγ to deg : Gain  Gain=180/pi
  aero scope : Scope
      settings: ShowLegends=on  YMin=-1000  YMax=6000  SaveName=ScopeData8
  aileron : Gain
  beta : Constant  Value=0
  canard : Gain
  coefficient : Subsystem
  cylindrical TF : Subsystem
  geometry(controller : Subsystem
  inertia(controller) : Subsystem
  limiter 143 deg below (5.3.3) : Saturate  UpperLimit=143 * pi / 180  LowerLimit=-143 * pi / 180
  mu_dot : Derivative
  pqr cmd Scope : Scope
      settings: SaveName=ScopeData2
  pqr cmd disp : Display
  pqr cmd to deg : Gain  Gain=180/pi
  pqr err Scope : Scope
      settings: SaveName=ScopeData4
  pqr err disp : Display
  pqr err to deg : Gain  Gain=180/pi
  rudder : Gain
  to deg1 : Gain  Gain=180/pi
  to rad2 : Gain  Commented=on  Gain=pi/180
  to rad3 : Gain  Gain=pi/180
  to rad4 : Gain  Gain=pi/180
  to rad5 : Gain  Commented=on  Gain=pi/180
  α cmd Scope : Scope
  α cmd disp : Display
  α_c to deg : Gain  Gain=180/pi
  αβμ err Scope : Scope
  αβμ err disp : Display
  αβμ err to deg : Gain  Gain=180/pi
  β_c to rad : Gain  Gain=pi/180
  γ : Terminator
  γ_c : Constant  Commented=on  Value=5
  μ γ calculator : Subsystem
  μ_dot_d Scope : Scope
      settings: SaveName=ScopeData3
  μ_dot_d disp : Display
  μ_dot_d to deg : Gain  Gain=180/pi
  ρ : Terminator
  χ_c : Constant  Commented=on  Value=5
  wires:
  Null flaps/1 -> Mux/4
  rudder/1 -> Mux/2
  canard/1 -> Mux/3
  Mux/1 -> IC/1
  IC/1 -> Model/1
  Clock/1 -> To Workspace x31control_time/1
  aileron/1 -> Mux/1
  Model/4 -> IC1/1
  Mux3/1 -> pqr cmd to deg/1, Mux8/2, Demux4/1, Sum1/1  "pqr command"
  Demux5/2 -> Sum1/2, Fast-State Controller pqr NDI/2(p q r)  "p q r"
  Fast-State Controller pqr NDI/3(canard) -> canard/1
  TVC z/1 -> Mux/6
  TVC y/1 -> Mux/7
  Fast-State Controller pqr NDI/1(aileron) -> aileron/1
  Fast-State Controller pqr NDI/2(rudder) -> rudder/1
  Fast-State Controller pqr NDI/4(TVC z) -> TVC z/1
  Fast-State Controller pqr NDI/5(TVC y) -> TVC y/1
  Sum2/1 -> Fast-State Controller pqr NDI/1(pqr dot desire)  "pqr dot desire"
  Demux3/3 -> PI Controller for r/1
  Demux3/2 -> PI Controller for q/1
  Demux3/1 -> PI Controller for p/1
  PI Controller for r/1 -> Mux1/3
  PI Controller for q/1 -> Mux1/2
  PI Controller for p/1 -> Mux1/1
  Mux1/1 -> Sum2/2
  Mux2/1 -> Sum2/1  "feedfoward"
  P gain for r/1 -> Mux2/3
  P gain for q/1 -> Mux2/2
  P gain for p/1 -> Mux2/1
  Demux4/1 -> P gain for p/1
  Demux4/2 -> P gain for q/1
  Demux4/3 -> P gain for r/1
  Model/2 -> Demux5/1  "Vxb Vyb Vzb p q r"
  Demux5/1 -> Term Vb/1
  coefficient/1(aero F) -> [X31controller_coef_F]
  coefficient/2(aero M) -> [X31controller_coef_M]
  [X31controller_coef_M] -> Fast-State Controller pqr NDI/4(coef M)
  geometry(controller/1(7 geo param(controller)) -> [X31controller_x31_geo]
  inertia(controller)/1(7 inertia param(controller)) -> [X31controller_x31_inertia]
  [X31controller_x31_geo] -> Fast-State Controller pqr NDI/5(geometry)
  [X31controller_x31_inertia] -> Fast-State Controller pqr NDI/6(inertia)
  Air density estimation/1(aeroV4) -> cylindrical TF/1(aeroV), Fast-State Controller pqr NDI/3(aero V), μ γ calculator/1(aero V4)  "aero V4"
  Slow-State Controller αβμ NDI/1(pc) -> Mux3/1
  Slow-State Controller αβμ NDI/2(qc) -> Mux3/2
  Slow-State Controller αβμ NDI/3(rc) -> Mux3/3
  Mux7/1 -> Demux2/1, Sum3/1  "α_c β_c μ_dot_c_lp"
  Sum3/1 -> αβμ err to deg/1, Demux1/1  "αβμ error"
  Demux1/3 -> I Controller for μ dot/1
  Demux1/2 -> PI Controller for β/1
  Demux1/1 -> PI Controller for α/1
  I Controller for μ dot/1 -> Mux4/3
  PI Controller for β/1 -> Mux4/2
  PI Controller for α/1 -> Mux4/1
  Mux4/1 -> Sum4/2
  Mux5/1 -> Sum4/1  "feedfoward"
  Demux2/3 -> P gain for μ/1  "(5.3.32)"
  P gain for β/1 -> Mux5/2
  P gain for α/1 -> Mux5/1
  Demux2/1 -> P gain for α/1
  Demux2/2 -> P gain for β/1
  Sum4/1 -> Slow-State Controller αβμ NDI/1(aero αβμ dot desire), Mux8/1
  Model/3 -> μ γ calculator/2(Q)  "Q0-Q3"
  [X31controller_coef_F] -> Slow-State Controller αβμ NDI/3(coef F)
  [X31controller_x31_geo] -> Slow-State Controller αβμ NDI/4(geometry)
  [X31controller_x31_inertia] -> Slow-State Controller αβμ NDI/5(inertia)
  Demux9/2 -> Slow-State Controller αβμ NDI/6(Thrust), Fast-State Controller pqr NDI/7(Thrust T)  "T, Ty, Tz"
  Mux6/1 -> Sum3/2  "α β μ_dot"
  Demux/2 -> Mux6/1
  Demux/4 -> mu_dot/1
  Demux/1 -> V/1
  Demux/5 -> γ/1
  Demux/3 -> ρ/1
  Maneuver generator/3 -> Mux11/3, μ_dot_d to deg/1, limiter 143 deg below (5.3.3)/1  "μ_dot_c"
  β_c to rad/1 -> Mux7/2  "β_c"
  Maneuver generator/2 -> Mux11/2, α_c to deg/1, Mux7/1  "α_c"
  beta/1 -> β_c to rad/1  "β_c"
  IC1/1 -> Air density estimation/1(aero V3)  "Vinf alpha beta"
  Demux9/1 -> Term cont/1
  Model/6 -> Demux9/1  "7controR, 7controlA, T, Ty, Tz"
  Mux10/1 -> To Workspace x31control_cmdVelAng/1, Sum5/1
  Sum5/1 -> Vχγ err Disp/1, Vχγ err Scope/1, Demux7/1  "Vχγ error"
  Demux7/3 -> PI Controller for γ/1
  Demux7/2 -> PI Controller for χ/1
  Demux7/1 -> PI Controller for V/1
  PI Controller for γ/1 -> Mux9/3
  PI Controller for χ/1 -> Mux9/2
  PI Controller for V/1 -> Mux9/1
  Model/1 -> Air density estimation/2(state X), IC4/1  "Vxe Vye Vze Xe   Ye   Ze"
  V_c/1 -> ?  "V_c"
  χ_c/1 -> ?  "Chi_c (χ_c)"
  γ_c/1 -> ?  "gamma_c (γ_c)"
  to rad3/1 -> Mux10/2
  to rad4/1 -> Mux10/3
  IC2/1 -> Demux/1, Maneuver generator/2, to deg1/1, coefficient/1(aug. aero)
  IC3/1 -> Sum5/2
  IC4/1 -> cylindrical TF/2(state X)
  mu_dot/1 -> Mux6/2
  P gain for μ/1 -> Mux5/3
  to deg1/1 -> V alpha beta rho mu gamma/1
  Thrust KN/1 -> Mux/5
  LPF for μ_dot/1 -> Mux7/3
  cylindrical TF/1(Vχγ) -> IC3/1, To Workspace x31control_stateVelAng/1, Vχγ to deg/1  "velocity angle"
  Vχγ to deg/1 -> Vχγ Scope/1
  μ γ calculator/1(aug. aeroV6) -> aero scope/1, To Workspace x31control_stateAeroAug/1, Slow-State Controller αβμ NDI/2(aug. aero V), IC2/1, AeroAug_dot/1  "V, α, β, ρ, μ, γ (rad)"
  [X31controller_x31_inertia] -> Maneuver generator/4
  [X31controller_x31_geo] -> Maneuver generator/3
  Mux9/1 -> Maneuver generator/1, Vχγ dot des scope/1, Vχγ dot des Disp/1  "Vχγ dot desire"
  Maneuver generator/1 -> Mux11/1, Thrust KN/1
  Mux11/1 -> To Workspace x31control_cmdAlpha/1
  α_c to deg/1 -> α cmd Scope/1, α cmd disp/1
  μ_dot_d to deg/1 -> μ_dot_d disp/1, μ_dot_d Scope/1
  αβμ err to deg/1 -> αβμ err disp/1, αβμ err Scope/1
  Sum1/1 -> Demux3/1, pqr err to deg/1  "pqr err"
  Mux8/1 -> To Workspace x31control_cmdAlpha1/1
  pqr cmd to deg/1 -> pqr cmd disp/1, pqr cmd Scope/1
  pqr err to deg/1 -> pqr err disp/1, pqr err Scope/1
  Model/5 -> Term IMU/1  "IMU"
  Signal Builder/1(Signal 1) -> to rad2/1
  Signal Builder/2(Signal 2) -> to rad5/1
  limiter 143 deg below (5.3.3)/1 -> LPF for μ_dot/1
  AeroAug_dot/1 -> To Workspace x31control_stateAeroAugDot/1
  Signal Builder1/3(Gamma) -> to rad4/1
  Signal Builder1/2(Chi) -> to rad3/1
  Signal Builder1/1(V) -> Mux10/1

== system X31dynamics_03_controller_NDI_MG/Air density estimation ==
  aero V3 : Inport
  state X : Inport  Port=2
  Mux : Mux  Inputs=2
  Terminator : Terminator
  air_density : Constant  Value=1.23
  aeroV4 : Outport
  wires:
  aero V3/1 -> Mux/1
  Mux/1 -> aeroV4/1
  air_density/1 -> Mux/2
  state X/1 -> Terminator/1

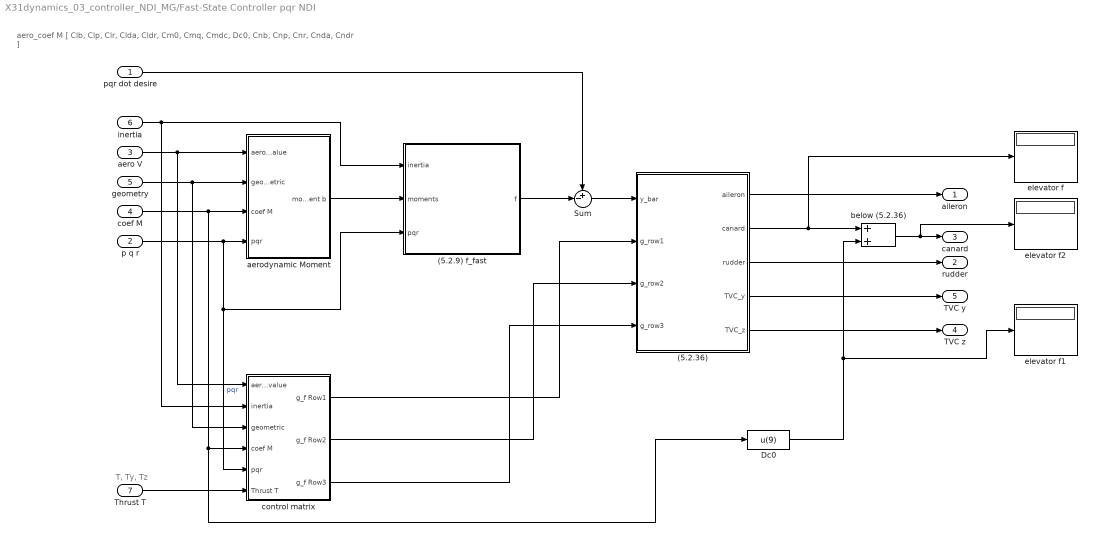
== system X31dynamics_03_controller_NDI_MG/Fast-State Controller pqr NDI ==
  note: aero_coef M
      | [ Clb, Clp, Clr, Clda, Cldr, Cm0, Cmq, Cmdc, Dc0, Cnb, Cnp, Cnr, Cnda, Cndr ]
  note: T, Ty, Tz
  pqr dot desire : Inport
  p q r : Inport  Port=2
  aero V : Inport  Port=3
  coef M : Inport  Port=4
  geometry : Inport  Port=5
  inertia : Inport  Port=6
  Thrust T : Inport  Port=7
  (5.2.36) : MATLAB Function  TreatAsAtomicUnit=on
  (5.2.9) f_fast : MATLAB Function  TreatAsAtomicUnit=on
  Dc0 : Fcn  Expr=u(9)
  Sum : Sum  Inputs=+-|
  aerodynamic Moment : Subsystem
  below (5.2.36) : Sum
  control matrix : Subsystem
  elevator f : Display
  elevator f1 : Display
  elevator f2 : Display
  aileron : Outport
  rudder : Outport  Port=2
  canard : Outport  Port=3
  TVC z : Outport  Port=4
  TVC y : Outport  Port=5
  wires:
  geometry/1 -> control matrix/3(geometric), aerodynamic Moment/2(geometric)
  coef M/1 -> Dc0/1, control matrix/4(coef M), aerodynamic Moment/3(coef M)
  aero V/1 -> control matrix/1(aero V value), aerodynamic Moment/1(aero V value)
  p q r/1 -> (5.2.9) f_fast/3(pqr), control matrix/5(pqr), aerodynamic Moment/4(pqr)  "pqr"
  aerodynamic Moment/1(moment b) -> (5.2.9) f_fast/2(moments)
  inertia/1 -> control matrix/2(inertia), (5.2.9) f_fast/1(inertia)
  Thrust T/1 -> control matrix/6(Thrust T)
  (5.2.9) f_fast/1(f) -> Sum/2
  pqr dot desire/1 -> Sum/1
  Sum/1 -> (5.2.36)/1(y_bar)
  (5.2.36)/1(aileron) -> aileron/1
  (5.2.36)/3(rudder) -> rudder/1
  (5.2.36)/2(canard) -> elevator f/1, below (5.2.36)/1
  (5.2.36)/5(TVC_z) -> TVC z/1
  (5.2.36)/4(TVC_y) -> TVC y/1
  control matrix/1(g_f Row1) -> (5.2.36)/2(g_row1)
  control matrix/2(g_f Row2) -> (5.2.36)/3(g_row2)
  control matrix/3(g_f Row3) -> (5.2.36)/4(g_row3)
  Dc0/1 -> elevator f1/1, below (5.2.36)/2
  below (5.2.36)/1 -> elevator f2/1, canard/1

== system X31dynamics_03_controller_NDI_MG/Signal Builder ==
  Demux : Demux  Tag=STV Demux  Outputs=3
  FromWs : FromWorkspace  Tag=STV FromWs  VariableName=tuvar  SampleTime=0
      SigBuilderData=|
      | common.afterFinalStr = 'Extrapolate'
      | common.sampleTime = 0
      | dataSet(1).timeRange = [0 30]
      | dataSet(1).name = 'Group 1'
      | dataSet(2).timeRange = [0 30]
      | dataSet(2).name = 'Group 2'
      | dataSet(3).timeRange = [0 30]
      | dataSet(3).name = 'Group 3'
      | dataSet(4).timeRange = [0 30]
      | dataSet(4).name = 'Group 4'
      | dataSet(5).timeRange = [0 30]
      | dataSet(5).name = 'Group 5'
      | sbobj.Groups(1).Name = 'Group 1'
      | sbobj.Groups(1).Signals(1).Name = 'Signal 1'
      | sbobj.Groups(1).Signals(1).XData = [0 5 5 25 25 30]
      | sbobj.Groups(1).Signals(1).YData = [10 10 30 30 10 10]
      | sbobj.Groups(1).Signals(2).Name = 'Signal 2'
      | sbobj.Groups(1).Signals(2).XData = [0 3 3 5 5 7 30]
      | sbobj.Groups(1).Signals(2).YData = [0 0 30 30 10 0 0]
      | sbobj.Groups(1).Signals(3).Name = 'Signal 3'
      | sbobj.Groups(1).Signals(3).XData = [0 1 1 20 20 30]
      | sbobj.Groups(1).Signals(3).YData = [80000 80000 120000 120000 80000 80000]
      | sbobj.Groups(1).TimeRange = [0 30]
      | sbobj.Groups(2).Name = 'Group 2'
      | sbobj.Groups(2).Signals(1).Name = 'Signal 1'
      | sbobj.Groups(2).Signals(1).XData = [0 4 15 30]
      | sbobj.Groups(2).Signals(1).YData = [-0.01 30 30 8.8]
      | sbobj.Groups(2).Signals(2).Name = 'Signal 2'
      | sbobj.Groups(2).Signals(2).XData = [0 0.625 1.25 1.875 2.5 3.125 3.75 4.375 5 5.625 6.25 6.875 7.5 8.125 8.75 9.375 10 10.625 11.25 11.875 12.5 13.125 13.75 14.375 15 15.625 16.25 16.875 17.5 18.125 18.75 19.375 20 20.625 21.25 21.875 22.5 23.125 23.75 24.375 25 25.625 26.25 26.875 27.5 28.125 28.75 29.375 30]
      | sbobj.Groups(2).Signals(2).YData = [0 14.1421356237 20 14.1421356237 2.44929359829e-15 -14.1421356237 -20 -14.1421356237 0 14.1421356237 20 14.1421356237 2.44929359829e-15 -14.1421356237 -20 -14.1421356237 0 14.1421356237 20 14.1421356237 2.44929359829e-15 -14.1421356237 -20 -14.1421356237 0 14.1421356237 20 14.1421356237 2.44929359829e-15 -14.1421356237 -20 -14.1421356237 0 14.1421356237 20 14.1421356237 2.44929359829e-15 -14.1421356237 -20 -14.1421356237 0 14.1421356237 20 14.1421356237 2.44929359829e-15 -14.1421356237 -20 -14.1421356237 0]
      | sbobj.Groups(2).Signals(3).Name = 'Signal 3'
      | sbobj.Groups(2).Signals(3).XData = [0 30]
      | sbobj.Groups(2).Signals(3).YData = [60 60]
      | sbobj.Groups(2).TimeRange = [0 30]
      | sbobj.Groups(3).Name = 'Group 3'
      | sbobj.Groups(3).Signals(1).Name = 'Signal 1'
      | sbobj.Groups(3).Signals(1).XData = [0 5 10 25 30]
      | sbobj.Groups(3).Signals(1).YData = [10 10 10 10 10]
      | sbobj.Groups(3).Signals(2).Name = 'Signal 2'
      | sbobj.Groups(3).Signals(2).XData = [0 3 3 9 9 30]
      | sbobj.Groups(3).Signals(2).YData = [0 0 30 30 0 0]
      | sbobj.Groups(3).Signals(3).Name = 'Signal 3'
      | sbobj.Groups(3).Signals(3).XData = [0 1 20 30]
      | sbobj.Groups(3).Signals(3).YData = [80000 80000 80000 80000]
      | sbobj.Groups(3).TimeRange = [0 30]
      | sbobj.Groups(4).Name = 'Group 4'
      | sbobj.Groups(4).Signals(1).Name = 'Signal 1'
      | sbobj.Groups(4).Signals(1).XData = [0 5 5 25 25 30]
      | sbobj.Groups(4).Signals(1).YData = [10 10 30 30 10 10]
      | sbobj.Groups(4).Signals(2).Name = 'Signal 2'
      | sbobj.Groups(4).Signals(2).XData = [0 3 3 8 8 9 30]
      | sbobj.Groups(4).Signals(2).YData = [0 0 30 30 10 0 0]
      | sbobj.Groups(4).Signals(3).Name = 'Signal 3'
      | sbobj.Groups(4).Signals(3).XData = [0 1 1 20 20 30]
      | sbobj.Groups(4).Signals(3).YData = [80000 80000 120000 120000 80000 80000]
      | sbobj.Groups(4).TimeRange = [0 30]
      | sbobj.Groups(5).Name = 'Group 5'
      | sbobj.Groups(5).Signals(1).Name = 'Signal 1'
      | sbobj.Groups(5).Signals(1).XData = [0 5 5 25 25 30]
      | sbobj.Groups(5).Signals(1).YData = [10 10 20 20 10 10]
      | sbobj.Groups(5).Signals(2).Name = 'Signal 2'
      | sbobj.Groups(5).Signals(2).XData = [0 3 3 5 5 7 30]
      | sbobj.Groups(5).Signals(2).YData = [0 0 30 30 10 0 0]
      | sbobj.Groups(5).Signals(3).Name = 'Signal 3'
      | sbobj.Groups(5).Signals(3).XData = [0 1 1 20 20 30]
      | sbobj.Groups(5).Signals(3).YData = [80000 80000 120000 120000 80000 80000]
      | sbobj.Groups(5).TimeRange = [0 30]
  Signal 1 : Outport  Tag=STV Outport
  Signal 2 : Outport  Tag=STV Outport  Port=2
  Signal 3 : Outport  Tag=STV Outport  Port=3
  wires:
  Demux/1 -> Signal 1/1
  FromWs/1 -> Demux/1
  Demux/2 -> Signal 2/1
  Demux/3 -> Signal 3/1

== system X31dynamics_03_controller_NDI_MG/Signal Builder1 ==
  Demux : Demux  Tag=STV Demux  Outputs=3
  FromWs : FromWorkspace  Tag=STV FromWs  VariableName=tuvar  SampleTime=0
      SigBuilderData=|
      | common.afterFinalStr = 'Extrapolate'
      | common.sampleTime = 0
      | dataSet.timeRange = [0 30]
      | dataSet.name = 'Group 5'
      | sbobj.Groups.Name = 'Group 5'
      | sbobj.Groups.Signals(1).Name = 'V'
      | sbobj.Groups.Signals(1).XData = [0 5 25 30]
      | sbobj.Groups.Signals(1).YData = [50 100 100 60]
      | sbobj.Groups.Signals(2).Name = 'Chi'
      | sbobj.Groups.Signals(2).XData = [0 2 8 15 25 29 30]
      | sbobj.Groups.Signals(2).YData = [0 5 60 -80 5 5 5]
      | sbobj.Groups.Signals(3).Name = 'Gamma'
      | sbobj.Groups.Signals(3).XData = [0 2 9 15 22 30]
      | sbobj.Groups.Signals(3).YData = [0 5 45 -45 0 5]
      | sbobj.Groups.TimeRange = [0 30]
  V : Outport  Tag=STV Outport
  Chi : Outport  Tag=STV Outport  Port=2
  Gamma : Outport  Tag=STV Outport  Port=3
  wires:
  Demux/1 -> V/1
  FromWs/1 -> Demux/1
  Demux/2 -> Chi/1
  Demux/3 -> Gamma/1

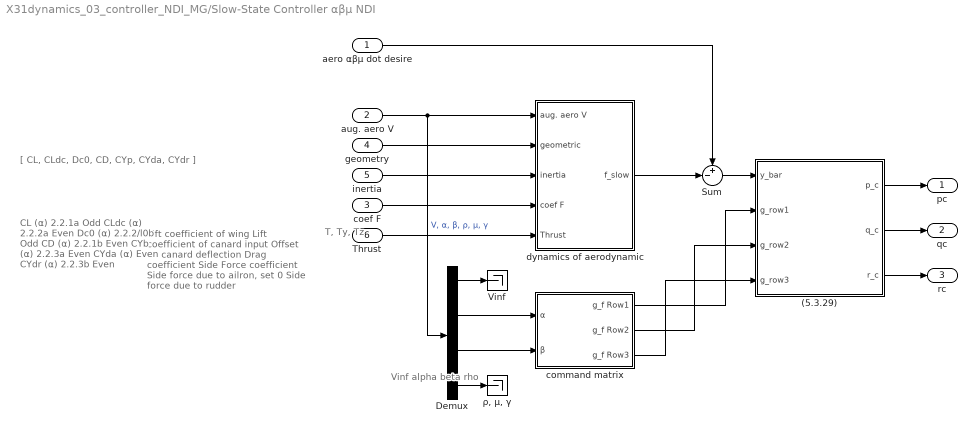
== system X31dynamics_03_controller_NDI_MG/Slow-State Controller αβμ NDI ==
  note: Vinf
      | alpha
      | beta
      | rho
  note: Lift coefficient of wing
      | Lift coefficient of canard input
      | Offset on canard deflection
      | Drag coefficient
      | Side Force coefficient
      | Side force due to ailron, set 0
      | Side force due to rudder
  note: CL     (α) 2.2.1a Odd
      | CLdc (α)  2.2.2a Even
      | Dc0   (α)  2.2.2/l0b Odd
      | CD     (α)  2.2.1b Even
      | CYb   (α) 2.2.3a Even
      | CYda (α)            Even
      | CYdr  (α) 2.2.3b Even
  note: [ CL, CLdc, Dc0, CD, CYp, CYda, CYdr ]
  note: T, Ty, Tz
  aero αβμ dot desire : Inport
  aug. aero V : Inport  Port=2
  coef F : Inport  Port=3
  geometry : Inport  Port=4
  inertia : Inport  Port=5
  Thrust : Inport  Port=6
  " ρ, μ, γ" : Terminator
  (5.3.29) : MATLAB Function  TreatAsAtomicUnit=on
  Demux : Demux  Outputs=[1 1 1 3]
  Sum : Sum  Inputs=+-|
  Vinf : Terminator
  command matrix : Subsystem
  dynamics of aerodynamic : Subsystem
  pc : Outport
  qc : Outport  Port=2
  rc : Outport  Port=3
  wires:
  geometry/1 -> dynamics of aerodynamic/2(geometric)
  coef F/1 -> dynamics of aerodynamic/4(coef F)
  inertia/1 -> dynamics of aerodynamic/3(inertia)
  dynamics of aerodynamic/1(f_slow) -> Sum/2
  aero αβμ dot desire/1 -> Sum/1
  Sum/1 -> (5.3.29)/1(y_bar)
  (5.3.29)/1(p_c) -> pc/1
  (5.3.29)/2(q_c) -> qc/1
  command matrix/1(g_f Row1) -> (5.3.29)/2(g_row1)
  command matrix/2(g_f Row2) -> (5.3.29)/3(g_row2)
  command matrix/3(g_f Row3) -> (5.3.29)/4(g_row3)
  aug. aero V/1 -> dynamics of aerodynamic/1(aug. aero V), Demux/1  "V, α, β, ρ, μ, γ"
  Thrust/1 -> dynamics of aerodynamic/5(Thrust)
  (5.3.29)/3(r_c) -> rc/1
  Demux/1 -> Vinf/1
  Demux/4 -> " ρ, μ, γ"/1
  Demux/2 -> command matrix/1(α)
  Demux/3 -> command matrix/2(β)

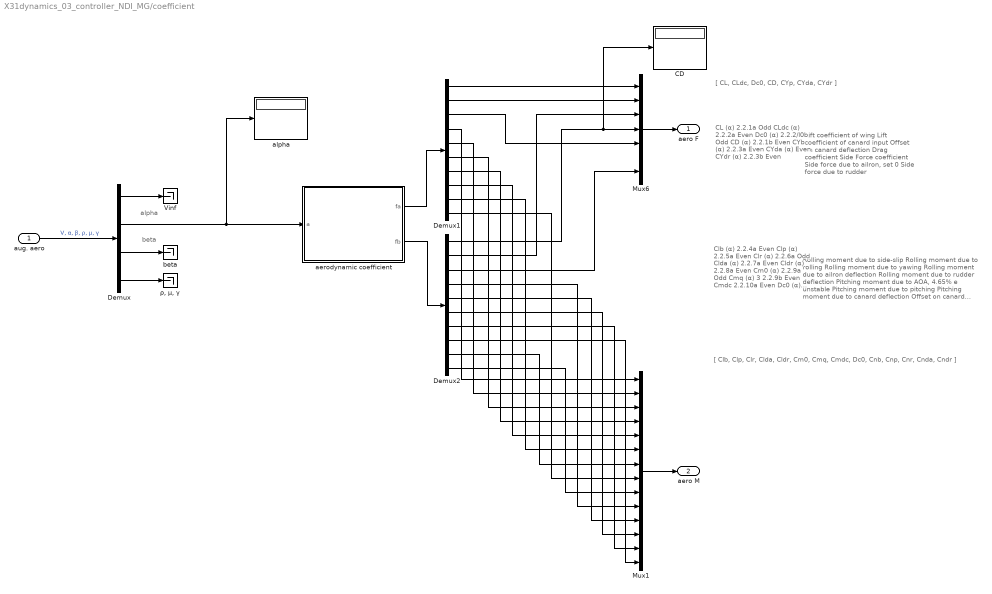
== system X31dynamics_03_controller_NDI_MG/coefficient ==
  note: Rolling moment due to side-slip
      | Rolling moment due to rolling
      | Rolling moment due to yawing
      | Rolling moment due to ailron deflection
      | Rolling moment due to rudder deflection
      |
      | Pitching moment due to AOA, 4.65% e unstable
      | Pitching moment due to pitching
      | Pitching moment due to canard deflection
      | Offset on canard deflection
      |
      | Yawing moment due to side-slip
      | Yawing moment due to rolling
      | Yawing moment due to yawing
      | Yawing moment due to ailron deflection
      | Yawing moment due to rudder deflection
  note: Lift coefficient of wing
      | Lift coefficient of canard input
      | Offset on canard deflection
      | Drag coefficient
      | Side Force coefficient
      | Side force due to ailron, set 0
      | Side force due to rudder
  note: Clb    (α) 2.2.4a Even
      | Clp    (α) 2.2.5a Even
      | Clr     (α) 2.2.6a Odd
      | Clda  (α) 2.2.7a Even
      | Cldr   (α) 2.2.8a Even
      |
      | Cm0  (α) 2.2.9a Odd
      | Cmq  (α) 3 2.2.9b Even
      | Cmdc      2.2.10a Even
      | Dc0   (α) 2.2.2/10b Odd
      |
      | Cnb  (α) 2.2.4b Even
      | Cnp  (α) 2.2.5b Odd
      | Cnr   (α) 2.2.6b Even
      | Cnda(α) 2.2.7b Even
      | Cndr (α) 2.2.8b Even
  note: CL     (α) 2.2.1a Odd
      | CLdc (α)  2.2.2a Even
      | Dc0   (α)  2.2.2/l0b Odd
      | CD     (α)  2.2.1b Even
      | CYb   (α) 2.2.3a Even
      | CYda (α)            Even
      | CYdr  (α) 2.2.3b Even
  note: beta
  note: alpha
  note: [ CL, CLdc, Dc0, CD, CYp, CYda, CYdr ]
  note: [ Clb, Clp, Clr, Clda, Cldr, Cm0, Cmq, Cmdc, Dc0, Cnb, Cnp, Cnr, Cnda, Cndr ]
  aug. aero : Inport
  CD : Display
  Demux : Demux  Outputs=[1 1 1 3]
  Demux1 : Demux  Outputs=10
  Demux2 : Demux  Outputs=10
  Mux1 : Mux  Inputs=14
  Mux6 : Mux  Inputs=7
  Vinf : Terminator
  aerodynamic coefficient : MATLAB Function  TreatAsAtomicUnit=on
  alpha : Display
  beta : Terminator
  "ρ, μ, γ" : Terminator
  aero F : Outport
  aero M : Outport  Port=2
  wires:
  Mux6/1 -> aero F/1
  aug. aero/1 -> Demux/1  "V, α, β, ρ, μ, γ"
  Demux/1 -> Vinf/1
  Mux1/1 -> aero M/1
  aerodynamic coefficient/1(fa) -> Demux1/1
  aerodynamic coefficient/2(fb) -> Demux2/1
  Demux1/1 -> Mux6/1
  Demux1/2 -> Mux6/2
  Demux2/2 -> Mux6/3
  Demux2/1 -> CD/1, Mux6/4
  Demux1/3 -> Mux6/5
  Demux2/3 -> Mux6/7
  Demux1/4 -> Mux1/1
  Demux1/5 -> Mux1/2
  Demux1/6 -> Mux1/3
  Demux1/7 -> Mux1/4
  Demux1/8 -> Mux1/5
  Demux1/9 -> Mux1/6
  Demux1/10 -> Mux1/8
  Demux2/4 -> Mux1/10
  Demux2/5 -> Mux1/11
  Demux2/6 -> Mux1/12
  Demux2/7 -> Mux1/13
  Demux2/8 -> Mux1/14
  Demux2/10 -> Mux1/9
  Demux2/9 -> Mux1/7
  Demux/3 -> beta/1
  Demux/2 -> alpha/1, aerodynamic coefficient/1(a)
  Demux/4 -> "ρ, μ, γ"/1

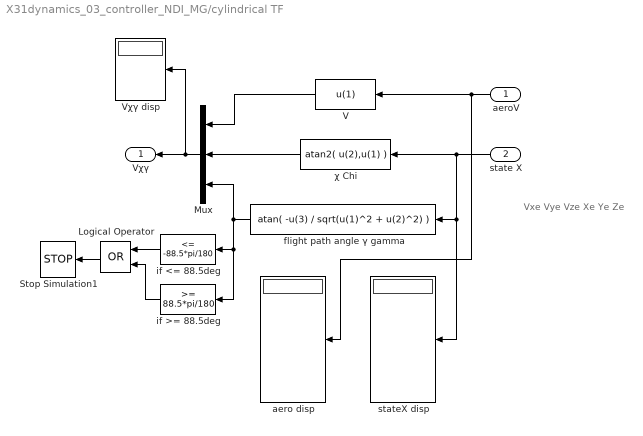
== system X31dynamics_03_controller_NDI_MG/cylindrical TF ==
  note: Vxe Vye Vze
      | Xe   Ye   Ze
  aeroV : Inport
  state X : Inport  Port=2
  Logical Operator : Logic  Operator=OR  AllPortsSameDT=off  OutDataTypeStr=boolean
  Mux : Mux  Inputs=3
  Stop Simulation1 : Stop
  V : Fcn  Expr=u(1)
  Vχγ disp : Display
  aero disp : Display
  flight path angle γ gamma : Fcn  Expr=atan( -u(3) / sqrt(u(1)^2 + u(2)^2) )
  if <= 88.5deg : simulink/Logic and Bit Operations/Compare To Constant  relop=<=  const=-88.5*pi/180  OutDataTypeStr=boolean
  if >= 88.5deg : simulink/Logic and Bit Operations/Compare To Constant  relop=>=  const=88.5*pi/180  OutDataTypeStr=boolean
  stateX disp : Display
  χ Chi : Fcn  Expr=atan2( u(2),u(1) )
  Vχγ : Outport
  wires:
  Mux/1 -> Vχγ disp/1, Vχγ/1
  aeroV/1 -> V/1, aero disp/1
  state X/1 -> stateX disp/1, flight path angle γ gamma/1, χ Chi/1
  V/1 -> Mux/1
  χ Chi/1 -> Mux/2
  flight path angle γ gamma/1 -> Mux/3, if >= 88.5deg/1, if <= 88.5deg/1
  if <= 88.5deg/1 -> Logical Operator/1
  if >= 88.5deg/1 -> Logical Operator/2
  Logical Operator/1 -> Stop Simulation1/1

== system X31dynamics_03_controller_NDI_MG/geometry(controller ==
  note: geometric
      |  [Sref, b, Cbar, Xp, Xc, Xr, Xt]
      |
      | Sref : reference wing area
      | b: Wing span
      | Cbar: Mean aerodynamic chord
      | Xp: pilot ahead of c.g.
      | Xc: Canard ahead of c.g.
      | Xr: Rudder aft of c.g.
      | Xt: Engine nozzle after of c.g.
  Cbar : Constant  Value=X31_controller.physical.geometry.Cbar
  Mux6 : Mux  Inputs=7
  Sref : Constant  Value=X31_controller.physical.geometry.Sref
  Xc : Constant  Value=X31_controller.physical.geometry.Xc
  Xp : Constant  Value=X31_controller.physical.geometry.Xp
  Xr : Constant  Value=X31_controller.physical.geometry.Xr
  Xt : Constant  Value=X31_controller.physical.geometry.Xt
  b : Constant  Value=X31_controller.physical.geometry.b
  7 geo param(controller) : Outport
  wires:
  Mux6/1 -> 7 geo param(controller)/1
  Sref/1 -> Mux6/1
  b/1 -> Mux6/2
  Cbar/1 -> Mux6/3
  Xp/1 -> Mux6/4
  Xc/1 -> Mux6/5
  Xr/1 -> Mux6/6
  Xt/1 -> Mux6/7

== system X31dynamics_03_controller_NDI_MG/inertia(controller) ==
  note: inetia
      | [m Ix Iy Iz Ixy Ixz Iyz]
      | m : mass
      | Ix Iy Iz Ixy Ixz Izy: rotational intertia
  Ix : Constant  Value=X31_controller.physical.inertia.Ixx
  Ixy : Constant  Value=X31_controller.physical.inertia.Ixy
  Ixz : Constant  Value=X31_controller.physical.inertia.Ixz
  Iy : Constant  Value=X31_controller.physical.inertia.Iyy
  Iyz : Constant  Value=X31_controller.physical.inertia.Iyz
  Iz : Constant  Value=X31_controller.physical.inertia.Izz
  Mux : Mux  Inputs=2
  Mux1 : Mux  Inputs=2
  Mux2 : Mux  Inputs=2
  Mux6 : Mux
  m : Constant  Value=X31_controller.physical.inertia.mass
  7 inertia param(controller) : Outport
  wires:
  Ix/1 -> Mux/1
  Iy/1 -> Mux/2
  Ixz/1 -> Mux2/1
  Iyz/1 -> Mux2/2
  Iz/1 -> Mux1/1
  Ixy/1 -> Mux1/2
  Mux6/1 -> 7 inertia param(controller)/1
  m/1 -> Mux6/1
  Mux/1 -> Mux6/2
  Mux1/1 -> Mux6/3
  Mux2/1 -> Mux6/4

== system X31dynamics_03_controller_NDI_MG/μ γ calculator ==
  aero V4 : Inport
  Q : Inport  Port=2
  -y : Gain  Gain=-1
  Body 2-3-1 to Q : QuaternionLib/Body 2-3-1 to Q
  Constant : Constant  Value=0
  Demux : Demux  Outputs=[1 1 1 1]
  Mux : Mux  Inputs=3
  Q to Body 3-2-1 get aero V eular : QuaternionLib/Q to Body 3-2-1
  Rho : Terminator
  Vinf : Terminator
  ground track angle : Terminator
  p rotiply q : QuaternionLib/p rotiply q
  aug. aeroV6 : Outport
  wires:
  Q/1 -> p rotiply q/2
  Demux/1 -> Vinf/1
  Demux/4 -> Rho/1
  Demux/2 -> -y/1  "α"
  Demux/3 -> Body 2-3-1 to Q/2  "β"
  aero V4/1 -> Mux/1, Demux/1
  -y/1 -> Body 2-3-1 to Q/1
  Constant/1 -> Body 2-3-1 to Q/3
  Body 2-3-1 to Q/1 -> p rotiply q/1
  p rotiply q/1 -> Q to Body 3-2-1 get aero V eular/1
  Mux/1 -> aug. aeroV6/1
  Q to Body 3-2-1 get aero V eular/1 -> ground track angle/1
  Q to Body 3-2-1 get aero V eular/2 -> Mux/3  "path angle γ"
  Q to Body 3-2-1 get aero V eular/3 -> Mux/2  "aero bank μ"

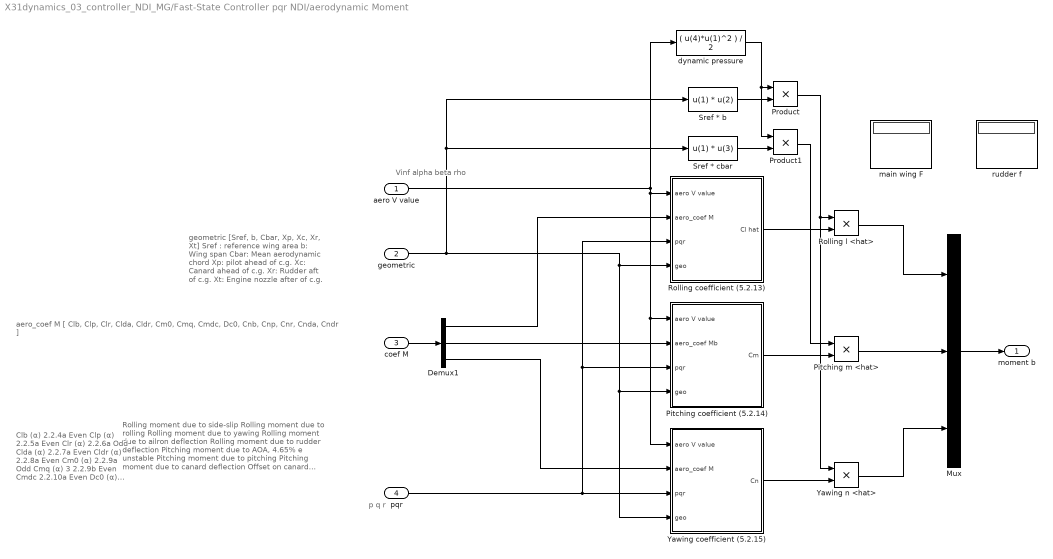
== system X31dynamics_03_controller_NDI_MG/Fast-State Controller pqr NDI/aerodynamic Moment ==
  note: Vinf alpha beta rho
  note: p q r
  note: geometric
      |  [Sref, b, Cbar, Xp, Xc, Xr, Xt]
      |
      | Sref : reference wing area
      | b: Wing span
      | Cbar: Mean aerodynamic chord
      | Xp: pilot ahead of c.g.
      | Xc: Canard ahead of c.g.
      | Xr: Rudder aft of c.g.
      | Xt: Engine nozzle after of c.g.
  note: Rolling moment due to side-slip
      | Rolling moment due to rolling
      | Rolling moment due to yawing
      | Rolling moment due to ailron deflection
      | Rolling moment due to rudder deflection
      |
      | Pitching moment due to AOA, 4.65% e unstable
      | Pitching moment due to pitching
      | Pitching moment due to canard deflection
      | Offset on canard deflection
      |
      | Yawing moment due to side-slip
      | Yawing moment due to rolling
      | Yawing moment due to yawing
      | Yawing moment due to ailron deflection
      | Yawing moment due to rudder deflection
  note: Clb    (α) 2.2.4a Even
      | Clp    (α) 2.2.5a Even
      | Clr     (α) 2.2.6a Odd
      | Clda  (α) 2.2.7a Even
      | Cldr   (α) 2.2.8a Even
      |
      | Cm0  (α) 2.2.9a Odd
      | Cmq  (α) 3 2.2.9b Even
      | Cmdc      2.2.10a Even
      | Dc0   (α) 2.2.2/10b Odd
      |
      | Cnb  (α) 2.2.4b Even
      | Cnp  (α) 2.2.5b Odd
      | Cnr   (α) 2.2.6b Even
      | Cnda(α) 2.2.7b Even
      | Cndr (α) 2.2.8b Even
  note: aero_coef M
      | [ Clb, Clp, Clr, Clda, Cldr, Cm0, Cmq, Cmdc, Dc0, Cnb, Cnp, Cnr, Cnda, Cndr ]
  aero V value : Inport
  geometric : Inport  Port=2
  coef M : Inport  Port=3
  pqr : Inport  Port=4
  Demux1 : Demux  Outputs=[5 4 5]
  Mux : Mux  Inputs=3
  Pitching coefficient (5.2.14) : Subsystem
  Pitching m <hat> : Product
  Product : Product
  Product1 : Product
  Rolling coefficient (5.2.13) : Subsystem
  Rolling l <hat> : Product
  Sref * b : Fcn  Expr=u(1) * u(2)
  Sref * cbar : Fcn  Expr=u(1) * u(3)
  Yawing coefficient (5.2.15) : Subsystem
  Yawing n <hat> : Product
  dynamic pressure : Fcn  Expr=( u(4)*u(1)^2 ) / 2
  main wing F : Display
  rudder f : Display
  moment b : Outport
  wires:
  Mux/1 -> moment b/1
  pqr/1 -> Rolling coefficient (5.2.13)/3(pqr), Pitching coefficient (5.2.14)/3(pqr), Yawing coefficient (5.2.15)/3(pqr)
  aero V value/1 -> Pitching coefficient (5.2.14)/1(aero V value), Yawing coefficient (5.2.15)/1(aero V value), Rolling coefficient (5.2.13)/1(aero V value), dynamic pressure/1
  Demux1/1 -> Rolling coefficient (5.2.13)/2(aero_coef M)
  coef M/1 -> Demux1/1
  Demux1/3 -> Yawing coefficient (5.2.15)/2(aero_coef M)
  Demux1/2 -> Pitching coefficient (5.2.14)/2(aero_coef Mb)
  geometric/1 -> Sref * b/1, Sref * cbar/1, Yawing coefficient (5.2.15)/4(geo), Pitching coefficient (5.2.14)/4(geo), Rolling coefficient (5.2.13)/4(geo)
  dynamic pressure/1 -> Product1/1, Product/1
  Sref * b/1 -> Product/2
  Product/1 -> Yawing n <hat>/1, Rolling l <hat>/1
  Rolling coefficient (5.2.13)/1(Cl hat) -> Rolling l <hat>/2
  Pitching coefficient (5.2.14)/1(Cm) -> Pitching m <hat>/2
  Yawing coefficient (5.2.15)/1(Cn) -> Yawing n <hat>/2
  Yawing n <hat>/1 -> Mux/3
  Rolling l <hat>/1 -> Mux/1
  Pitching m <hat>/1 -> Mux/2
  Sref * cbar/1 -> Product1/2
  Product1/1 -> Pitching m <hat>/1
